simulink model "model_LOC3"  (R2021b)
settings: Solver=VariableStepAuto  StartTime=0.0  StopTime=T  RelTol=1e-3
settings Model: Creator=mateusz  LastModifiedBy=mateusz

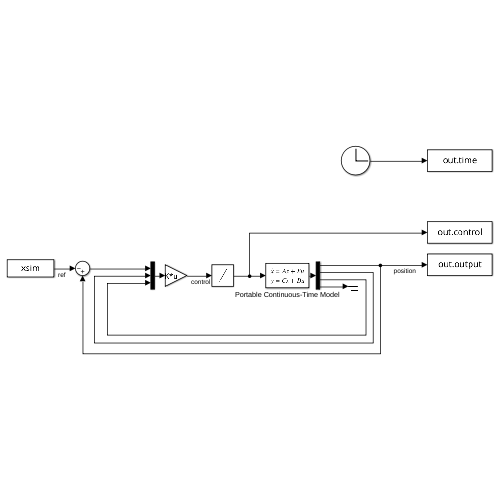
[thumbnail: Simulink's stored preview of the top-level diagram]
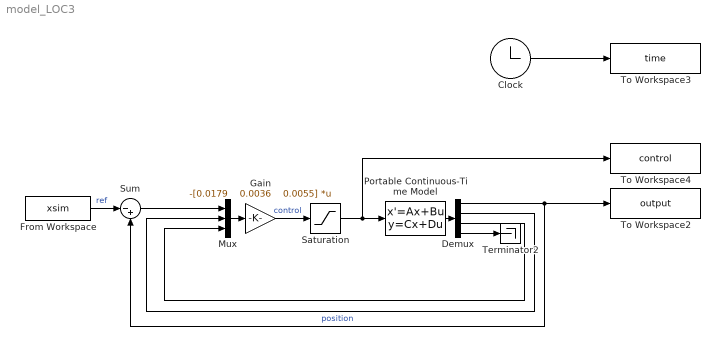
== system model_LOC3 ==
  Clock : Clock
  Demux : Demux
  From Workspace : FromWorkspace  VariableName=xsim
  Gain : Gain  Gain="-[0.0179    0.0036    0.0055]"  Multiplication=Matrix(K*u)
  Mux : Mux  Inputs=3
  Portable Continuous-Time Model : StateSpace  A=|  B=[0;0;0;2.59e4];  C=eye(4,4)  D=zeros(4,1)  InitialCondition=0
      | [0  1  0    0;
      |      0 -5  4.5  0;
      |      0  0 -0.7108*2  23.6012*2;
      |      0  0 -5.3898 -4040];
  Saturation : Saturate
  Sum : Sum  Inputs=|-+
  Terminator2 : Terminator
  To Workspace2 : ToWorkspace  VariableName=output  SampleTime=0.02
  To Workspace3 : ToWorkspace  VariableName=time  SampleTime=0.02
  To Workspace4 : ToWorkspace  VariableName=control  SampleTime=0.02
  wires:
  Portable Continuous-Time Model/1 -> Demux/1
  Demux/3 -> Mux/3
  Demux/4 -> Terminator2/1
  Clock/1 -> To Workspace3/1
  Demux/2 -> Mux/2
  Demux/1 -> To Workspace2/1, Sum/2  "position"
  Gain/1 -> Saturation/1  "control"
  From Workspace/1 -> Sum/1  "ref"
  Saturation/1 -> To Workspace4/1, Portable Continuous-Time Model/1
  Mux/1 -> Gain/1
  Sum/1 -> Mux/1
